simulink model "chap2_3sim"  (Simulink 7.7)
settings: Solver=ode45  StartTime=0.0  StopTime=15  RelTol=1e-3
settings Model: Creator=ljk  LastModifiedBy=ljk  ExtModeTrigMode=oneshot  ExtModeArmWhenConnect=off
settings DataIOCC: LimitDataPoints=off  SignalLoggingName=sigsOut
settings OptimizationCC: BooleanDataType=off
settings DebuggingCC: SaveWithParameterizedLinksMsg=none  SignalResolutionControl=TryResolveAllWithWarning  SolverPrmCheckMsg=none  MultiTaskDSMMsg=warning  MultiTaskCondExecSysMsg=none  StrictBusMsg=None
settings HardwareCC: TargetUnknown=on
settings RTWCC: IncludeERTFirstTime=on

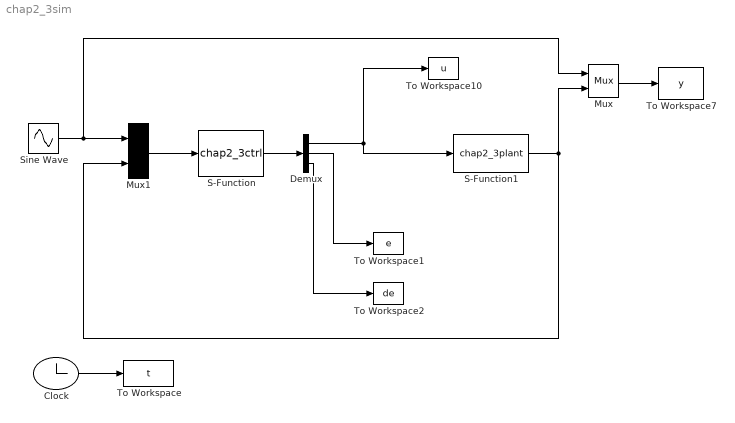
== system chap2_3sim ==
  Clock : Clock
  Demux : Demux  Outputs=3
  Mux : Mux  Inputs=2
  Mux1 : Mux  Inputs=2
  S-Function : S-Function  FunctionName=chap2_3ctrl  EnableBusSupport=off
  S-Function1 : S-Function  FunctionName=chap2_3plant  EnableBusSupport=off
  Sine Wave : Sin  SampleTime=0
  To Workspace : ToWorkspace  VariableName=t  SampleTime=-1  SaveFormat=Array
  To Workspace1 : ToWorkspace  VariableName=e  SampleTime=-1  SaveFormat=Array
  To Workspace10 : ToWorkspace  VariableName=u  SampleTime=-1  SaveFormat=Array
  To Workspace2 : ToWorkspace  VariableName=de  SampleTime=-1  SaveFormat=Array
  To Workspace7 : ToWorkspace  VariableName=y  SampleTime=-1  SaveFormat=Array
  wires:
  Sine Wave/1 -> Mux/1, Mux1/1
  Mux1/1 -> S-Function/1
  Clock/1 -> To Workspace/1
  Mux/1 -> To Workspace7/1
  S-Function1/1 -> Mux/2, Mux1/2
  S-Function/1 -> Demux/1
  Demux/1 -> To Workspace10/1, S-Function1/1
  Demux/2 -> To Workspace1/1
  Demux/3 -> To Workspace2/1
